simulink model "Longitudinal_MPC_Control2020b"  (R2020b)
settings: Solver=VariableStepAuto  StartTime=0.0  StopTime=60  RelTol=1e-3
settings Model: Creator=PC  LastModifiedBy=lenovo
settings DebuggingCC: SFMachineParentedDataDiag=error

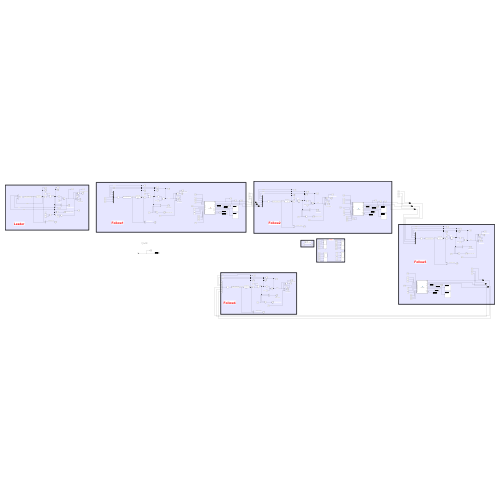
[thumbnail: Simulink's stored preview of the top-level diagram]
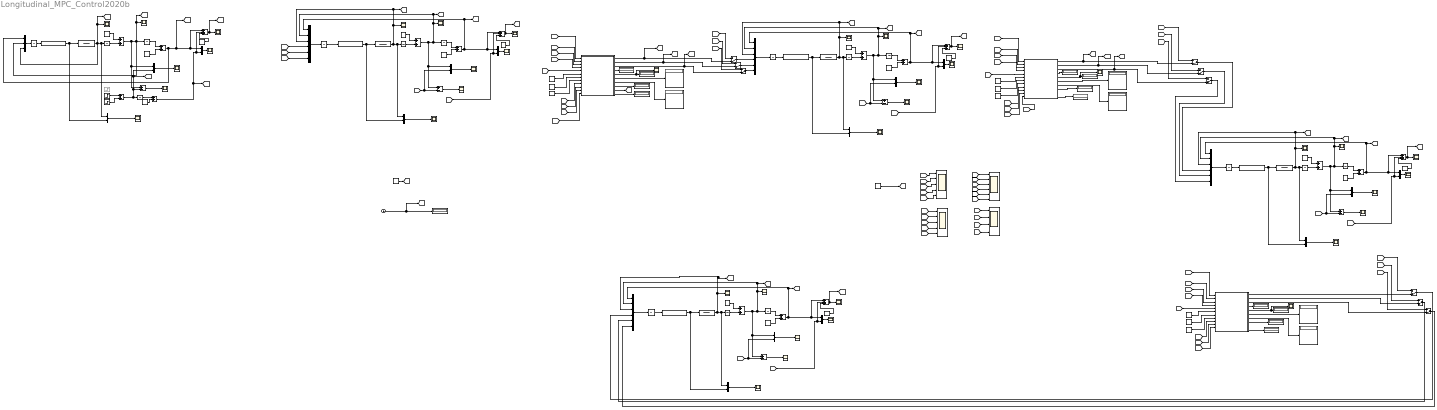
== system Longitudinal_MPC_Control2020b ==
  note: 结果输出
  note: 带宽确认参数
  note: 当前带宽确认参数
      | aerfa=0：busy
      | aerfa=1：idle
      | aerfa（0，1）：moderate
  note: 期望速度和实际速度之间的偏差
  note: 实际加速度
  note: 期望加速度
  note: 被控对象传递函数
  note: 实际速度
  note: 初始位置
  note: 实际位置和leader位置
  note: 初始速度
  note: lesder速度/期望速度和实际速度
  note: 期望加速度和实际加速度
  note: 实际位置和期望位置之间的偏差
  note: 实际位置和期望位置之间的偏差
  note: 期望速度和实际速度之间的偏差
  note: 被控对象传递函数
  note: 期望加速度
  note: 初始位置
  note: 实际速度
  note: 实际位置和期望位置
  note: 初始速度
  note: 实际加速度
  note: 期望速度和实际速度
  note: 期望加速度和实际加速度
  note: 实际速度
  note: 实际加速度
  note: 实际位置
  note: 实际位置
  note: 实际位置
  note: 实际速度
  note: 实际位置
  note: 实际加速度
  note: 实际位置和期望位置之间的偏差
  note: 期望速度和实际速度之间的偏差
  note: 期望加速度和实际加速度
  note: 实际加速度
  note: 初始位置
  note: 实际位置和期望位置
  note: 期望速度和实际速度
  note: 实际速度
  note: 被控对象传递函数
  note: 初始速度
  note: 期望加速度
  note: 实际位置和期望位置之间的偏差
  note: 被控对象传递函数
  note: 实际加速度
  note: 实际位置
  note: 实际位置
  note: 实际加速度
  note: 期望速度和实际速度
  note: 实际速度
  note: 期望速度和实际速度之间的偏差
  note: 初始位置
  note: 期望加速度和实际加速度
  note: 实际位置和期望位置
  note: 初始速度
  note: 期望加速度
  note: 实际速度
  note: 实际位置和期望位置之间的偏差
  note: 被控对象传递函数
  note: 实际加速度
  note: 实际位置
  note: 实际位置
  note: 实际加速度
  note: 期望速度和实际速度
  note: 实际速度
  note: 期望速度和实际速度之间的偏差
  note: 初始位置
  note: 期望加速度和实际加速度
  note: 实际位置和期望位置
  note: 初始速度
  note: 期望加速度
  note: 实际速度
  note: 实际加速度
  note: 实际速度
  note: 实际位置
  note: Leader
  note: Follow1
  note: Follow2
  note: Follow3
  note: Follow4
  Bus Creator : BusCreator  Inputs=3
  Bus Creator{1..3,5..7,9..13,15..17,19} (15 alike) : BusCreator  Inputs=2
  Bus Creator{4,8,14,18} (4 alike) : BusCreator  Inputs=6
  Clock : Clock
  Display{,1..18} (19 alike) : Display
  Follow1_a : TransferFcn  Denominator=[0.5 1]
  Follow1_e : Sum  Inputs=+-+
  Follow1_p : Sum
  Follow1_v : Sum
  Follow2_a : TransferFcn  Denominator=[0.5 1]
  Follow2_e : Sum  Inputs=+-+
  Follow2_p : Sum
  Follow2_v : Sum
  Follow3_a : TransferFcn  Denominator=[0.5 1]
  Follow3_e : Sum  Inputs=+-+
  Follow3_p : Sum
  Follow3_v : Sum
  Follow4_a : TransferFcn  Denominator=[0.5 1]
  Follow4_e : Sum  Inputs=+-+
  Follow4_p : Sum
  Follow4_v : Sum
  Integrator{1..11} (11 alike) : Integrator
  Leader_a : TransferFcn  Denominator=[0.5 1]
  Leader_e : Sum  Inputs=+-+
  Leader_p : Sum
  Leader_v : Sum
  MATLAB Function1 : MATLAB Function  TreatAsAtomicUnit=on
  MATLAB Function2 : MATLAB Function  TreatAsAtomicUnit=on
  MATLAB Function3 : MATLAB Function  TreatAsAtomicUnit=on
  Manual Switch{,1..8} (9 alike) : ManualSwitch  CurrentSetting=0
  Ref_v : Sum
  S-Function : S-Function  Priority=1  FunctionName=Car1_MPC_Longitudinal_Control  SFunctionDeploymentMode=off  EnableBusSupport=off
  S-Function1 : S-Function  Priority=2  FunctionName=Car2_MPC_Longitudinal_Control  SFunctionDeploymentMode=off  EnableBusSupport=off
  S-Function2 : S-Function  Priority=3  FunctionName=Car3_MPC_Longitudinal_Control  SFunctionDeploymentMode=off  EnableBusSupport=off
  S-Function3 : S-Function  Priority=4  FunctionName=Car4_MPC_Longitudinal_Control  SFunctionDeploymentMode=off  EnableBusSupport=off
  S-Function4 : S-Function  Priority=5  FunctionName=Car5_MPC_Longitudinal_Control  SFunctionDeploymentMode=off  EnableBusSupport=off
  Scope : Scope
  Scope1 : Scope
  Scope2 : Scope
  Step : Step  Commented=on  Before=3  After=5  SampleTime=0
  Step1 : Step  Time=8  Before=3  After=6  SampleTime=0
  Step3 : Step  Time=24  After=-2  SampleTime=0
  Unit Delay{,1..4} (5 alike) : UnitDelay  SampleTime=-1  HasFrameUpgradeWarning=on
  V00 : Constant  Value=3
  V{1..4} (4 alike) : Constant  Value=3
  X{1..2,4,6,9} (5 alike) : Sum  Inputs=+-
  X3 : Sum
  u{1..21,26..39} (35 alike) : Scope
  u22 : Scope  NumInputPorts=5
  u23 : Scope  NumInputPorts=6
  u24 : Scope  NumInputPorts=5
  u25 : Scope  NumInputPorts=4
  x1 : Constant  Value=40
  x10 : Constant  Value=0
  x{3,5,7..9,11} (6 alike) : Constant  Value=10
  x12 : Constant  Value=0.5
  x{13..22} (10 alike) : Constant
  x2 : Constant  Value=50
  x4 : Constant  Value=30
  x6 : Constant  Value=20
  wires:
  S-Function/1 -> Bus Creator2/2, Leader_a/1
  Leader_a/1 -> Bus Creator/3, [a1], u8/1, Bus Creator2/1, Integrator2/1
  Integrator2/1 -> Leader_v/2
  V00/1 -> Leader_v/1
  Leader_v/1 -> Bus Creator1/1, X2/1, Bus Creator/2, Integrator3/1, u7/1, [v1]
  Integrator3/1 -> Leader_p/1
  x1/1 -> Leader_p/2
  Leader_p/1 -> [p1], Leader_e/1, Bus Creator3/1, Bus Creator/1
  X2/1 -> u1/1
  Bus Creator1/1 -> u2/1
  Bus Creator2/1 -> u3/1
  Bus Creator3/1 -> u5/1
  Integrator4/1 -> X3/1
  x2/1 -> X3/2
  X3/1 -> Leader_e/2, Bus Creator3/2, [p0]
  Leader_e/1 -> [e1], u4/1
  x3/1 -> Leader_e/3
  [p1] -> Follow1_e/2, Bus Creator7/2
  Bus Creator7/1 -> u12/1
  Follow1_e/1 -> [e2], u11/1
  Bus Creator4/1 -> Unit Delay1/1
  x4/1 -> Follow1_p/2
  Follow1_a/1 -> u14/1, Bus Creator4/3, [a2], Bus Creator6/1, Integrator7/1
  Follow1_p/1 -> Follow1_e/1, Bus Creator7/1, Bus Creator4/1, [p2]
  Integrator8/1 -> Follow1_p/1
  Bus Creator5/1 -> u9/1
  V1/1 -> Follow1_v/1
  X6/1 -> u6/1
  S-Function1/1 -> Bus Creator6/2, Follow1_a/1
  Follow1_v/1 -> Bus Creator5/1, X6/1, Bus Creator4/2, [v2], u13/1, Integrator8/1
  Bus Creator6/1 -> u10/1
  Integrator7/1 -> Follow1_v/2
  Unit Delay1/1 -> S-Function1/1
  [v1] -> Bus Creator5/2, X6/2
  x5/1 -> Follow1_e/3
  Follow2_v/1 -> X9/1, Bus Creator9/1, Bus Creator8/2, [v3], u18/1, Integrator9/1
  Unit Delay2/1 -> S-Function2/1
  [p2] -> Follow2_e/2, Bus Creator11/2
  Bus Creator10/1 -> u15/1
  [v2] -> Bus Creator9/2, X9/2
  Follow2_e/1 -> [e3], u16/1
  Bus Creator11/1 -> u17/1
  S-Function2/1 -> Bus Creator10/2, Follow2_a/1
  X9/1 -> u20/1
  Follow2_a/1 -> u19/1, Bus Creator8/3, [a3], Bus Creator10/1, Integrator6/1
  x7/1 -> Follow2_e/3
  x6/1 -> Follow2_p/2
  Bus Creator8/1 -> Unit Delay2/1
  Integrator6/1 -> Follow2_v/2
  Bus Creator9/1 -> u21/1
  Integrator9/1 -> Follow2_p/1
  V2/1 -> Follow2_v/1
  Follow2_p/1 -> Follow2_e/1, Bus Creator11/1, Bus Creator8/1, [p3]
  [v3] -> u23/4
  [v0] -> u23/1
  [v2] -> u23/3
  [v1] -> u23/2
  [e3] -> u25/2
  [e2] -> u25/1
  x9/1 -> Follow3_e/3
  Follow3_a/1 -> u30/1, Bus Creator14/3, [a4], Bus Creator12/1, Integrator1/1
  x8/1 -> Follow3_p/2
  Follow3_e/1 -> [e4], u27/1
  Bus Creator15/1 -> u32/1
  Follow3_p/1 -> Follow3_e/1, Bus Creator13/1, Bus Creator14/1, [p4]
  S-Function3/1 -> Bus Creator12/2, Follow3_a/1
  Integrator5/1 -> Follow3_p/1
  V3/1 -> Follow3_v/1
  Bus Creator14/1 -> Unit Delay3/1
  Integrator1/1 -> Follow3_v/2
  Bus Creator13/1 -> u28/1
  Bus Creator12/1 -> u26/1
  [p3] -> Follow3_e/2, Bus Creator13/2
  X1/1 -> u31/1
  [v3] -> Bus Creator15/2, X1/2
  Unit Delay3/1 -> S-Function3/1
  Follow3_v/1 -> Bus Creator15/1, X1/1, Bus Creator14/2, [v4], u29/1, Integrator5/1
  x11/1 -> Follow4_e/3
  Follow4_a/1 -> u37/1, Bus Creator18/3, [a5], Bus Creator16/1, Integrator10/1
  x10/1 -> Follow4_p/2
  Follow4_e/1 -> [e5], u34/1
  Bus Creator19/1 -> u39/1
  Follow4_p/1 -> Follow4_e/1, Bus Creator17/1, Bus Creator18/1, [p5]
  S-Function4/1 -> Bus Creator16/2, Follow4_a/1
  Integrator11/1 -> Follow4_p/1
  V4/1 -> Follow4_v/1
  Bus Creator18/1 -> Unit Delay4/1
  Integrator10/1 -> Follow4_v/2
  Bus Creator17/1 -> u35/1
  Bus Creator16/1 -> u33/1
  [p4] -> Follow4_e/2, Bus Creator17/2
  X4/1 -> u38/1
  [v4] -> Bus Creator19/2, X4/2
  Unit Delay4/1 -> S-Function4/1
  Follow4_v/1 -> Bus Creator19/1, X4/1, Bus Creator18/2, [v5], u36/1, Integrator11/1
  [p1] -> u22/1
  [p2] -> u22/2
  [p3] -> u22/3
  [p4] -> u22/4
  [p5] -> u22/5
  [v5] -> u23/6
  [v4] -> u23/5
  [e4] -> u25/3
  [e5] -> u25/4
  Clock/1 -> [time_s], Display/1
  x12/1 -> [aerfa]
  x13/1 -> [a0]
  [a1] -> u24/1
  [a2] -> u24/2
  [a3] -> u24/3
  [a4] -> u24/4
  [a5] -> u24/5
  Step1/1 -> Ref_v/1
  Step3/1 -> Ref_v/2
  Ref_v/1 -> X2/2, Bus Creator1/2, [v0], Integrator4/1
  Bus Creator/1 -> Unit Delay/1
  Unit Delay/1 -> S-Function/1
  [time_s] -> MATLAB Function1/1(t)
  [aerfa] -> MATLAB Function1/5(aerfa)
  [p1] -> Bus Creator4/4
  [v1] -> Bus Creator4/5
  [a1] -> Bus Creator4/6
  [p2] -> MATLAB Function1/2(p2)
  [v2] -> MATLAB Function1/3(v2)
  [a2] -> MATLAB Function1/4(a2)
  x14/1 -> MATLAB Function1/6(yo12)
  x15/1 -> MATLAB Function1/7(yo22)
  x16/1 -> MATLAB Function1/8(yo32)
  [p1] -> MATLAB Function1/9(p1)
  [v1] -> MATLAB Function1/10(v1)
  [a1] -> MATLAB Function1/11(a1)
  MATLAB Function1/4(f_2) -> Display1/1
  MATLAB Function1/5(flag2) -> Scope/1, Display2/1
  MATLAB Function1/6(error1_2) -> Display3/1
  MATLAB Function1/7(error2_2) -> Display4/1
  MATLAB Function1/8(sgma_2) -> Display5/1
  Manual Switch/1 -> Bus Creator8/4
  Manual Switch1/1 -> Bus Creator8/5
  Manual Switch2/1 -> Bus Creator8/6
  [p2] -> Manual Switch/1
  [v2] -> Manual Switch1/1
  [a2] -> Manual Switch2/1
  MATLAB Function1/1(pp2) -> [pp2], Manual Switch/2
  MATLAB Function1/2(vv2) -> [vv2], Manual Switch1/2
  MATLAB Function1/3(aa2) -> [aa2], Manual Switch2/2
  MATLAB Function1/10(tri_2) -> Display6/1
  MATLAB Function2/10(tri_3) -> Display12/1
  MATLAB Function2/1(pp3) -> [pp3], Manual Switch3/2
  MATLAB Function2/3(aa3) -> [aa3], Manual Switch5/2
  MATLAB Function2/2(vv3) -> [vv3], Manual Switch4/2
  x19/1 -> MATLAB Function2/8(yo33)
  [time_s] -> MATLAB Function2/1(t)
  MATLAB Function2/5(flag3) -> Scope1/1, Display8/1
  MATLAB Function2/8(sgma_3) -> Display11/1
  [p3] -> MATLAB Function2/2(p3)
  [a3] -> MATLAB Function2/4(a3)
  MATLAB Function2/7(F_3) -> Display10/1
  MATLAB Function2/4(f_3) -> Display7/1
  [v3] -> MATLAB Function2/3(v3)
  x17/1 -> MATLAB Function2/6(yo13)
  x18/1 -> MATLAB Function2/7(yo23)
  [p2] -> MATLAB Function2/9(pp2)
  MATLAB Function2/6(E_3) -> Display9/1
  [aerfa] -> MATLAB Function2/5(aerfa)
  [p3] -> Manual Switch3/1
  [v3] -> Manual Switch4/1
  [a3] -> Manual Switch5/1
  Manual Switch3/1 -> Bus Creator14/4
  Manual Switch4/1 -> Bus Creator14/5
  Manual Switch5/1 -> Bus Creator14/6
  MATLAB Function3/2(vv4) -> Manual Switch7/2
  [aerfa] -> MATLAB Function3/5(aerfa)
  [pp3] -> MATLAB Function3/9(pp3)
  [vv3] -> MATLAB Function3/10(vv3)
  MATLAB Function3/6(E_4) -> Display18/1
  x21/1 -> MATLAB Function3/7(yo24)
  MATLAB Function3/7(F_4) -> Display13/1
  [aa3] -> MATLAB Function3/11(aa3)
  [p4] -> MATLAB Function3/2(p4)
  MATLAB Function3/5(flag4) -> Scope2/1, Display17/1
  MATLAB Function3/4(f_4) -> Display16/1
  MATLAB Function3/8(sgma_4) -> Display14/1
  [a4] -> MATLAB Function3/4(a4)
  [v4] -> MATLAB Function3/3(v4)
  x20/1 -> MATLAB Function3/6(yo14)
  MATLAB Function3/3(aa4) -> Manual Switch8/2
  x22/1 -> MATLAB Function3/8(yo34)
  MATLAB Function3/10(tri_4) -> Display15/1
  MATLAB Function3/1(pp4) -> Manual Switch6/2
  [time_s] -> MATLAB Function3/1(t)
  [v4] -> Manual Switch7/1
  [a4] -> Manual Switch8/1
  [p4] -> Manual Switch6/1
  Manual Switch6/1 -> Bus Creator18/4
  Manual Switch7/1 -> Bus Creator18/5
  Manual Switch8/1 -> Bus Creator18/6
  [vv2] -> MATLAB Function2/10(vv2)
  [aa2] -> MATLAB Function2/11(aa2)
  MATLAB Function1/9(xx02) -> [xx02]
  [xx02] -> MATLAB Function2/12(xx02)
  [p0] -> MATLAB Function1/12(p0)

== matlab function Longitudinal_MPC_Control2020b/MATLAB Function1 ==
  settings: updateMethod=DISCRETE
  data: t input; p2 input; v2 input; a2 input; aerfa input; yo12 input; yo22 input; yo32 input; pp2 output; p1 input; v1 input; a1 input; vv2 output; aa2 output; f_2 output; flag2 output; error1_2 output; error2_2 output; sgma_2 output; xx02 output; tri_2 output; p0 input
function [pp2,vv2,aa2,f_2,flag2,error1_2,error2_2,sgma_2,xx02,tri_2]  = event_trigger2(t,p2,v2,a2,aerfa,yo12,yo22,yo32,p1,v1,a1,p0)
%% 偏差是上次传输时刻的状态-当前采样时刻的状态
%fai是位置偏差、速度偏差、加速度偏差的权重
persistent x02 sgmai101 sgmai201 k_2 trigger2 t02 px02 count2;
if isempty(x02)
    x02=zeros(3,1);%上一时刻传输的状态量,不包含位置
    x02=[0;3;0];
    px02=zeros(3,1);%上一时刻传输的状态量,包含位置
    px02=[30;3;0];
    count2=0;
    t02=0;%事件触发时刻时间记忆
    sgmai101=0.1;%自适应参数初始化
    sgmai201=1.1;%自适应参数初始化
    k_2=1;%触发时刻计数变量
    trigger2=zeros(100000,1);
end
flag2=0;
x1_2=zeros(3,1);
x1_2=[p2;v2;a2];%本车的状态信息
x1_20=[0;v2;a2];
x1_0=[p1;v1;a1];%前一辆车的传输状态,leader默认时刻传输
ds1=0.01/v2;%速度大的时候，为了保证传输加快，则系数应该变小.单纯设计为0.008也可以
error1_2=px02-x1_2+x1_0-x1_2-[10;0;0];%上次触发时刻状态与当前状态之间的偏差，代表车辆2参考状态的转移/位置有问题+跟踪前车传输的状态的误差
error2_2=[ds1/(px02(1)-x1_0(1));ds1/(px02(2)-x1_0(2));ds1/(px02(3)-x1_0(3))];
% psai_1=[1,20,10];%触发条件中的误差权重向量，增大pasi，增大f
fai_1=[yo12,yo22,yo32];%增大fai，减小f
psai_1=fai_1;
%求解触发条件自适应参数
E_1=norm((psai_1.^0.5)*error1_2)*norm((psai_1.^0.5)*error1_2);
F_1=norm((fai_1.^0.5)*error2_2)*norm((fai_1.^0.5)*error2_2);
%原参数
ri1_1=0.001;
ri2_1=0.0000005;
sgmai_min=0.01;
sgmai_max=1.2;

%新参数
% ri1_1=0.008;
% ri2_1=0.000000002;
% sgmai_min=0.35;
% sgmai_max=0.56;

sgmai1_1=sgmai101/(1+ri1_1*sgmai101*E_1);
sgmai2_1=(sgmai201*E_1+ri2_1*sgmai_max)/(ri2_1+E_1);
sgma_2=sgmai1_1*aerfa+(1-aerfa)*sgmai2_1;%求解触发条件自适应参数

%%触发条件
f_2=E_1-sgma_2*F_1;
if f_2>0  %%事件触发
    pp2=p2;
    vv2=v2;
    aa2=a2;
    x02=x1_20;%不包含位置信息
    px02=x1_2;%包含位置信息
    trigger2(k_2)=t;
    k_2=k_2+1;
    t02=t;
    flag2=1;
    count2=count2+1;
else
    pp2=px02(1)+(t-t02)*px02(2);
    vv2=px02(2)+(t-t02)*px02(3);
    aa2=px02(3);
    flag2=0;%事件不触发
end
xx02=px02;
tri_2=count2;
% tri_1=trigger2;
end

== matlab function Longitudinal_MPC_Control2020b/MATLAB Function2 ==
  settings: updateMethod=DISCRETE
  data: t input; p3 input; v3 input; a3 input; aerfa input; yo13 input; yo23 input; yo33 input; pp3 output; pp2 input; vv3 output; aa3 output; f_3 output; flag3 output; E_3 output; F_3 output; sgma_3 output; xx03 output; tri_3 output; vv2 input; aa2 input; xx02 input
function [pp3,vv3,aa3,f_3,flag3,E_3,F_3,sgma_3,xx03,tri_3]  = event_trigger3(t,p3,v3,a3,aerfa,yo13,yo23,yo33,pp2,vv2,aa2,xx02)
%% 偏差是上次传输时刻的状态-当前采样时刻的状态
%fai是位置偏差、速度偏差、加速度偏差的权重
persistent x03 sgmai103 sgmai203 k_3 trigger3 t03 px03 count3;
if isempty(x03)
    x03=zeros(3,1);
    px03=zeros(3,1);
    x03=[0;3;0];
    px03=[20;3;0];
    count3=0;
    t03=0;%事件触发时刻时间记忆
    sgmai103=0.1;%自适应参数初始化
    sgmai203=1.1;%自适应参数初始化
    k_3=1;%触发时刻计数变量
    trigger3=zeros(100000,1);
end
flag3=0;
x1_3=zeros(3,1);
x1_3=[p3;v3;a3];%本车的状态信息
x2_0=[pp2;vv2;aa2];%前一辆车的传输状态,leader默认时刻传输

ds3=0.01/v3;
error1_3=px03-x1_3+x2_0-x1_3-[10;0;0];%上次触发时刻状态与当前状态之间的偏差，代表车辆2参考状态的转移/位置有问题
error2_3=[ds3/(px03(1)-x2_0(1));ds3/(px03(2)-x2_0(2));ds3/(px03(3)-x2_0(3))];%车辆1的上一时刻触发状态与车辆0触发状态之间的偏差，代表跟随精确程度
fai_3=[yo13,yo23,yo33];%增大fai，减小f
psai_3=fai_3;
%求解触发条件自适应参数
E_3=norm((psai_3.^0.5)*error1_3)*norm((psai_3.^0.5)*error1_3);
F_3=norm((fai_3.^0.5)*error2_3)*norm((fai_3.^0.5)*error2_3);
%原参数
ri1_3=0.001;
ri2_3=0.0000005;
sgmai_min=0.01;
sgmai_max=1.2;


sgmai1_3=sgmai103/(1+ri1_3*sgmai103*E_3);
sgmai2_3=(sgmai203*E_3+ri2_3*sgmai_max)/(ri2_3+E_3);
sgma_3=sgmai1_3*aerfa+(1-aerfa)*sgmai2_3;%求解触发条件自适应参数

%%触发条件
f_3=E_3-sgma_3*F_3;
if f_3>0  %%事件触发
    pp3=p3;
    vv3=v3;
    aa3=a3;
    px03=x1_3;%包含位置信息
    trigger3(k_3)=t;
    k_3=k_3+1;
    t03=t;
    flag3=1;
    count3=count3+1;
else
    pp3=px03(1)+(t-t03)*px03(2);
    vv3=px03(2)+(t-t03)*px03(3);
    aa3=px03(3);
    flag3=0;%事件不触发
end
xx03=px03;
tri_3=count3;
end

== matlab function Longitudinal_MPC_Control2020b/MATLAB Function3 ==
  settings: updateMethod=DISCRETE
  data: t input; p4 input; v4 input; a4 input; aerfa input; yo14 input; yo24 input; yo34 input; pp4 output; pp3 input; vv3 input; aa3 input; vv4 output; aa4 output; f_4 output; flag4 output; E_4 output; F_4 output; sgma_4 output; xx04 output; tri_4 output
function [pp4,vv4,aa4,f_4,flag4,E_4,F_4,sgma_4,xx04,tri_4]  = event_trigger4(t,p4,v4,a4,aerfa,yo14,yo24,yo34,pp3,vv3,aa3)
%% 偏差是上次传输时刻的状态-当前采样时刻的状态
%fai是位置偏差、速度偏差、加速度偏差的权重
persistent x04 sgmai104 sgmai204 k_4 trigger4 t04 px04 count4;
if isempty(x04)
    x04=zeros(3,1);%上一时刻传输的状态量,不包含位置
    px04=zeros(3,1);%上一时刻传输的状态量,包含位置
    px04=[10;3;0];
    count4=0;
    t04=0;%事件触发时刻时间记忆
    sgmai104=0.1;%自适应参数初始化
    sgmai204=1.1;%自适应参数初始化
    k_4=1;%触发时刻计数变量
    trigger4=zeros(100000,1);
end
flag4=0;
x1_4=zeros(3,1);
x1_4=[p4;v4;a4];%本车的状态信息
x3_0=[pp3;vv3;aa3];%前一辆车的传输状态,leader默认时刻传输
error1_4=px04-x1_4+x3_0-x1_4-[10;0;0];%上次触发时刻状态与当前状态之间的偏差，代表车辆2参考状态的转移/位置有问题
ds4=0.01/v4;
error2_4=[ds4/(px04(1)-x3_0(1));ds4/(px04(2)-x3_0(2));ds4/(px04(3)-x3_0(3))];%车辆1的上一时刻触发状态与车辆0触发状态之间的偏差，代表跟随精确程度
fai_4=[yo14,yo24,yo34];%增大fai，减小f
psai_4=fai_4;
%求解触发条件自适应参数
E_4=norm((psai_4.^0.5)*error1_4)*norm((psai_4.^0.5)*error1_4);
F_4=norm((fai_4.^0.5)*error2_4)*norm((fai_4.^0.5)*error2_4);
%原参数
ri1_4=0.001;
ri2_4=0.0000005;
sgmai_min=0.01;
sgmai_max=1.2;

sgmai1_4=sgmai104/(1+ri1_4*sgmai104*E_4);
sgmai2_4=(sgmai204*E_4+ri2_4*sgmai_max)/(ri2_4+E_4);
sgma_4=sgmai1_4*aerfa+(1-aerfa)*sgmai2_4;%求解触发条件自适应参数

%%触发条件
f_4=E_4-sgma_4*F_4;
if f_4>0  %%事件触发
    pp4=p4;
    vv4=v4;
    aa4=a4;
    px04=x1_4;%包含位置信息
    trigger4(k_4)=t;
    k_4=k_4+1;
    t04=t;
    flag4=1;
    count4=count4+1;
else
    pp4=px04(1)+(t-t04)*px04(2);
    vv4=px04(2)+(t-t04)*px04(3);
    aa4=px04(3);
    flag4=0;%事件不触发
end
xx04=px04;
tri_4=count4;
end
